simulink subsystem "RangoTheta"  (R2020a)
settings: Solver=VariableStepAuto  StartTime=0.0  StopTime=10.0  RelTol=1e-3
settings Model: Creator=charlie  LastModifiedBy=charlie

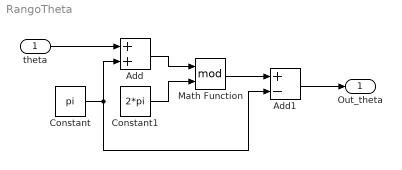
== system RangoTheta ==
  theta : Inport
  Add : Sum
  Add1 : Sum  Inputs=+-
  Constant : Constant  Value=pi
  Constant1 : Constant  Value=2*pi
  Math Function : Math  Operator=mod  SaturateOnIntegerOverflow=on
  Out_theta : Outport
  wires:
  theta/1 -> Add/1
  Add/1 -> Math Function/1
  Constant/1 -> Add1/2, Add/2
  Add1/1 -> Out_theta/1
  Constant1/1 -> Math Function/2
  Math Function/1 -> Add1/1
